simulink model "Y_Delta_Connected"  (R2018a)
settings: Solver=VariableStepAuto  StartTime=0.0  StopTime=stopTime  FixedStep=1e-8  MaxStep=1e-7  RelTol=1e-3
values from neighbouring files (symbols this model uses):
  Cp = 1/(res_w^2*Lp)    [design_code.m]
  Cs = 1/(res_w^2*Ls)    [design_code.m]
  fop = 155    [param.m]
  M = 10^6*M    [design_code.m]    (also in param.m = [p1 p1p2 p1p3 p1s1 p1s2 p1s3 ;      p1p2 p2 p2p3 p2s1 p2s2 p)
  R = [3 0 0 0 0 0 ... (first row only)    [param.m]
  R_L = Vout^2/P_o    [design_code.m]
  Vin_peak = (100)*sqrt(2)    [param.m]
libraries: powerlib x50, pePowerMeasurement x2, powerlib_meascontrol x1
settings Model: Creator=enes_  LastModifiedBy=enes_
settings SolverCC: ZeroCrossAlgorithm=Adaptive
settings DebuggingCC: MaxConsecutiveZCsMsg=none

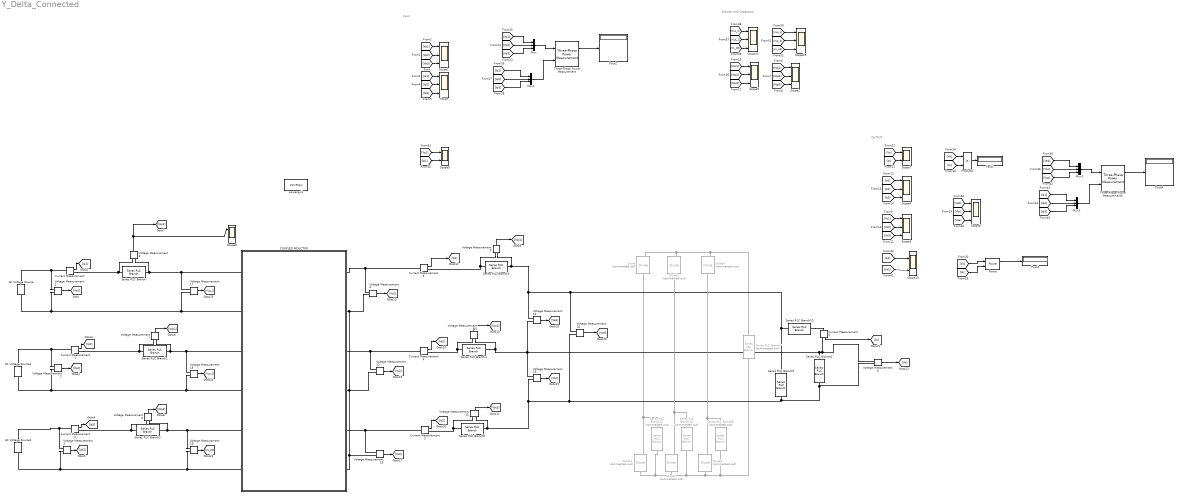
== system Y_Delta_Connected ==
  note: Inductor and Capacitors
  note: OUTPUT
  note: Input
  AC Voltage Source : powerlib/Electrical Sources/AC Voltage Source  Amplitude=Vin_peak  Phase=0  Frequency=fop*1e3  SampleTime=0  Measurements=None  BusType=swing  Pref=10e3  Qref=0  Qmin=-inf  Qmax=+inf
  AC Voltage Source1 : powerlib/Electrical Sources/AC Voltage Source  Amplitude=Vin_peak  Phase=120  Frequency=fop*1e3  SampleTime=0  Measurements=None  BusType=swing  Pref=10e3  Qref=0  Qmin=-inf  Qmax=+inf
  AC Voltage Source2 : powerlib/Electrical Sources/AC Voltage Source  Amplitude=Vin_peak  Phase=240  Frequency=fop*1e3  SampleTime=0  Measurements=None  BusType=swing  Pref=10e3  Qref=0  Qmin=-inf  Qmax=+inf
  COUPLED INDUCTOR : Subsystem
  Current Measurement{,1..6} (7 alike) : powerlib/Measurements/Current Measurement  PhasorSimulation=off  OutputType=Complex  PSBequivalent=0
  Diode{,1..5} (6 alike) : powerlib/Power Electronics/Diode  Commented=on  Ron=0.001  Lon=0  Vf=0.8  IC=0  UseSnubber=0  Rs=inf  Cs=250e-9  Measurements=on
  Mux{,1..3} (4 alike) : Mux  Inputs=3
  Pout{1..4} (4 alike) : Display
  Power : powerlib_meascontrol/Measurements/Power  Freq=fop*1e3  Vinit=[1, 0]  Iinit=[1, 0]  Ts=0
      settings: SourceProductName=Simscape Power Systems
  Product4 : Product
  Scope{,1..6,11,15} (9 alike) : Scope  NumInputPorts=3
  Scope{7..9,13} (4 alike) : Scope  NumInputPorts=2
  Series RLC Branch : powerlib/Elements/Series RLC Branch  LConnTagsString=__new0  RConnTagsString=__new0  BranchType=C  Resistance=1  Inductance=1e-3  SetiL0=off  InitialCurrent=0  Capacitance=Cp  Setx0=off  InitialVoltage=0  Measurements=None
  Series RLC Branch1 : powerlib/Elements/Series RLC Branch  LConnTagsString=__new0  RConnTagsString=__new0  BranchType=C  Resistance=1  Inductance=1e-3  SetiL0=off  InitialCurrent=0  Capacitance=Cp  Setx0=off  InitialVoltage=0  Measurements=None
  Series RLC Branch10 : powerlib/Elements/Series RLC Branch  LConnTagsString=__new0  RConnTagsString=__new0  BranchType=R  Resistance=R_L  Inductance=1e-3  SetiL0=off  InitialCurrent=0  Capacitance=9.95e-9  Setx0=off  InitialVoltage=0  Measurements=None
  Series RLC Branch15 : powerlib/Elements/Series RLC Branch  Commented=on  LConnTagsString=__new0  RConnTagsString=__new0  BranchType=R  Resistance=1e5  Inductance=1e-3  SetiL0=off  InitialCurrent=0  Capacitance=9.95e-9  Setx0=off  InitialVoltage=0  Measurements=None
  Series RLC Branch16 : powerlib/Elements/Series RLC Branch  Commented=on  LConnTagsString=__new0  RConnTagsString=__new0  BranchType=R  Resistance=1e5  Inductance=1e-3  SetiL0=off  InitialCurrent=0  Capacitance=9.95e-9  Setx0=off  InitialVoltage=0  Measurements=None
  Series RLC Branch2 : powerlib/Elements/Series RLC Branch  LConnTagsString=__new0  RConnTagsString=__new0  BranchType=C  Resistance=1  Inductance=1e-3  SetiL0=off  InitialCurrent=0  Capacitance=Cp  Setx0=off  InitialVoltage=0  Measurements=None
  Series RLC Branch3 : powerlib/Elements/Series RLC Branch  LConnTagsString=__new0  RConnTagsString=__new0  BranchType=C  Resistance=1  Inductance=1e-3  SetiL0=off  InitialCurrent=0  Capacitance=Cs  Setx0=off  InitialVoltage=0  Measurements=None
  Series RLC Branch4 : powerlib/Elements/Series RLC Branch  LConnTagsString=__new0  RConnTagsString=__new0  BranchType=C  Resistance=1  Inductance=1e-3  SetiL0=off  InitialCurrent=0  Capacitance=Cs  Setx0=off  InitialVoltage=0  Measurements=None
  Series RLC Branch5 : powerlib/Elements/Series RLC Branch  LConnTagsString=__new0  RConnTagsString=__new0  BranchType=C  Resistance=1  Inductance=1e-3  SetiL0=off  InitialCurrent=0  Capacitance=Cs  Setx0=off  InitialVoltage=0  Measurements=None
  Series RLC Branch6 : powerlib/Elements/Series RLC Branch  LConnTagsString=__new0  RConnTagsString=__new0  BranchType=R  Resistance=R_L  Inductance=1e-3  SetiL0=off  InitialCurrent=0  Capacitance=9.95e-9  Setx0=off  InitialVoltage=0  Measurements=None
  Series RLC Branch7 : powerlib/Elements/Series RLC Branch  Commented=on  LConnTagsString=__new0  RConnTagsString=__new0  BranchType=C  Resistance=30  Inductance=1e-3  SetiL0=off  InitialCurrent=0  Capacitance=1e-6  Setx0=off  InitialVoltage=0  Measurements=None
  Series RLC Branch8 : powerlib/Elements/Series RLC Branch  Commented=on  LConnTagsString=__new0  RConnTagsString=__new0  BranchType=R  Resistance=1e5  Inductance=1e-3  SetiL0=off  InitialCurrent=0  Capacitance=9.95e-9  Setx0=off  InitialVoltage=0  Measurements=None
  Series RLC Branch9 : powerlib/Elements/Series RLC Branch  LConnTagsString=__new0  RConnTagsString=__new0  BranchType=R  Resistance=R_L  Inductance=1e-3  SetiL0=off  InitialCurrent=0  Capacitance=9.95e-9  Setx0=off  InitialVoltage=0  Measurements=None
  Three-Phase Power Measurement : pePowerMeasurement/Three-Phase Power Measurement  OverrideUsingVariant=Continuous  F=fop*1e3  K=1  Seq=Negative  Ts=0
  Three-Phase Power Measurement1 : pePowerMeasurement/Three-Phase Power Measurement  OverrideUsingVariant=Continuous  F=fop*1e3  K=1  Seq=Negative  Ts=0
  Voltage Measurement{1..19} (19 alike) : powerlib/Measurements/Voltage Measurement  PhasorSimulation=off  OutputType=Complex  PSBequivalent=0
  powergui1 : powerlib/powergui  Priority=1  SimulationMode=Continuous  SampleTime=50e-6  frequency=60  Iterations=50  frequencyindice=155000  Pbase=100e6  ErrMax=1e-4  UnitsV=kV  UnitsW=MW  buscounter=0  FunctionMessages=off  echomessages=off  EnableUseOfTLC=off  CurrentSourceSwitches=off  DisableSnubberDevices=off  DisableRonSwitches=off  DisableVfSwitches=off  DisplayEquations=off  SolverType=Tustin/Backward Euler (TBE)  Interpol=off  ExternalGateDelay=off  methode=off  Ts=100  x0status=blocks  SPID=on  SwTol=0  HookPort=off  RestoreLinks=warning  ResistiveCurrentMeasurement=off  Frange=[0:2:500]  Ylog=off  Xlog=on  ShowGrid=off  save=off  variable=ZData  structure=0  ZoomFFT=off  StartTime=0.0  cycles=1  DisplayStyle=1  fundamental=60  FreqAxis=off  MaxFrequency=1000  frequencyindicesteady=1  RmsSteady=1  display=off
  wires:
  [VLp_2] -> Scope15/2
  [VL_p3] -> Scope15/3
  Voltage Measurement3/1 -> [Vp3]
  [Vsc3] -> Scope5/3
  Voltage Measurement19/1 -> [VL_p3]
  [Vsc2] -> Scope5/2
  Voltage Measurement13/1 -> [Vs3]
  [Vcp2] -> Scope2/2
  [Vcp3] -> Scope2/3
  Voltage Measurement2/1 -> [Vp2]
  [Ip2] -> Scope/2
  Voltage Measurement17/1 -> [VLp_1]
  Current Measurement2/1 -> [Ip3]
  Voltage Measurement7/1 -> [Vcp2]
  Current Measurement/1 -> [Ip1]
  [Vp1] -> Scope9/1
  [VLp_2] -> Scope11/1
  Voltage Measurement18/1 -> [VLp_2]
  Voltage Measurement11/1 -> [Vsc3]
  [Vsc1] -> Scope5/1
  [Is3] -> Scope4/3
  [VL_p3] -> Scope11/3
  Current Measurement5/1 -> [Is1]
  [Vcp1] -> Scope2/1
  [Io] -> Scope7/2
  Voltage Measurement14/1 -> [Vab]
  [Is2] -> Scope4/2
  [Vp2] -> Scope1/2
  [Vs3] -> Scope3/3
  [Vp1] -> Scope1/1
  [Vs2] -> Scope3/2
  [Vp3] -> Scope1/3
  [Vs1] -> Scope3/1
  [Ip1] -> Scope/1
  [Vo] -> Scope7/1
  Voltage Measurement9/1 -> [Vsc1]
  Current Measurement1/1 -> [Ip2]
  Voltage Measurement1/1 -> [Vp1]
  [Is1] -> Scope4/1
  [Ip3] -> Scope/3
  Voltage Measurement10/1 -> [Vsc2]
  [Ip1] -> Scope9/2
  Voltage Measurement5/1 -> [Vcp3]
  [VLp_1] -> Scope11/2
  Current Measurement4/1 -> [Is2]
  Voltage Measurement6/1 -> [Vo]
  Current Measurement3/1 -> [Is3]
  Voltage Measurement16/1 -> [Vca]
  Current Measurement6/1 -> [Io]
  Voltage Measurement12/1 -> [Vs2]
  Voltage Measurement8/1 -> Scope8/1, [Vcp1]
  Voltage Measurement4/1 -> [Vs1]
  Voltage Measurement15/1 -> [Vbc]
  [VLp_1] -> Scope15/1
  [Is1] -> Scope13/1
  [Vs1] -> Scope13/2
  [Io] -> Product4/2
  [Vo] -> Product4/1
  Product4/1 -> Pout1/1
  [Vp1] -> Mux/1
  [Vp2] -> Mux/2
  [Vp3] -> Mux/3
  [Ip2] -> Mux1/2
  [Ip1] -> Mux1/1
  [Ip3] -> Mux1/3
  Mux1/1 -> Three-Phase Power Measurement/2
  Mux/1 -> Three-Phase Power Measurement/1
  Three-Phase Power Measurement/1 -> Pout2/1
  [Vab] -> Scope6/1
  [Vca] -> Scope6/3
  [Vbc] -> Scope6/2
  [Vo] -> Power/1
  [Io] -> Power/2
  Power/1 -> Pout3/1
  [Ip1] -> Mux3/1
  [Ip3] -> Mux3/3
  [Vbc] -> Mux2/2
  [Ip2] -> Mux3/2
  [Vab] -> Mux2/1
  Mux3/1 -> Three-Phase Power Measurement1/2
  [Vca] -> Mux2/3
  Mux2/1 -> Three-Phase Power Measurement1/1
  Three-Phase Power Measurement1/1 -> Pout4/1
  connections:
  Current Measurement/LConn1 -- Voltage Measurement1/LConn1 -- AC Voltage Source/RConn1
  Diode2/RConn1 -- Series RLC Branch7/LConn1 -- Diode4/RConn1 -- Diode/RConn1
  Current Measurement4/LConn1 -- COUPLED INDUCTOR/LConn3 -- Voltage Measurement12/LConn1
  Current Measurement5/LConn1 -- Voltage Measurement4/LConn1 -- COUPLED INDUCTOR/LConn1
  Series RLC Branch/RConn1 -- Voltage Measurement8/LConn2 -- COUPLED INDUCTOR/RConn1 -- Voltage Measurement17/LConn1
  Series RLC Branch8/RConn1 -- Series RLC Branch7/RConn1 -- Series RLC Branch15/RConn1 -- Diode3/LConn1 -- Series RLC Branch16/RConn1 -- Diode1/LConn1 -- Diode5/LConn1
  Series RLC Branch4/LConn1 -- Current Measurement4/RConn1 -- Voltage Measurement10/LConn1
  Series RLC Branch1/RConn1 -- Voltage Measurement7/LConn2 -- COUPLED INDUCTOR/RConn3 -- Voltage Measurement18/LConn1
  Series RLC Branch2/LConn1 -- Current Measurement2/RConn1 -- Voltage Measurement5/LConn1
  AC Voltage Source2/RConn1 -- Current Measurement2/LConn1 -- Voltage Measurement3/LConn1
  Current Measurement1/LConn1 -- Voltage Measurement2/LConn1 -- AC Voltage Source1/RConn1
  Voltage Measurement4/LConn2 -- Voltage Measurement12/LConn2 -- COUPLED INDUCTOR/LConn4 -- Voltage Measurement13/LConn2 -- COUPLED INDUCTOR/LConn6 -- COUPLED INDUCTOR/LConn2
  Diode/LConn1 -- Series RLC Branch16/LConn1 -- Diode1/RConn1
  Series RLC Branch2/RConn1 -- COUPLED INDUCTOR/RConn5 -- Voltage Measurement19/LConn1 -- Voltage Measurement5/LConn2
  Series RLC Branch1/LConn1 -- Current Measurement1/RConn1 -- Voltage Measurement7/LConn1
  Series RLC Branch6/LConn1 -- Voltage Measurement6/LConn1 -- Current Measurement6/RConn1 -- Voltage Measurement15/LConn1 -- Voltage Measurement14/LConn2 -- Voltage Measurement10/LConn2 -- Series RLC Branch4/RConn1
  Series RLC Branch/LConn1 -- Current Measurement/RConn1 -- Voltage Measurement8/LConn1
  Series RLC Branch6/RConn1 -- Voltage Measurement16/LConn1 -- Series RLC Branch5/RConn1 -- Voltage Measurement11/LConn2 -- Voltage Measurement15/LConn2 -- Series RLC Branch9/RConn1 -- Voltage Measurement6/LConn2
  Series RLC Branch3/LConn1 -- Current Measurement5/RConn1 -- Voltage Measurement9/LConn1
  Current Measurement3/RConn1 -- Series RLC Branch5/LConn1 -- Voltage Measurement11/LConn1
  AC Voltage Source1/LConn1 -- COUPLED INDUCTOR/RConn4 -- Voltage Measurement18/LConn2 -- Voltage Measurement2/LConn2
  Voltage Measurement17/LConn2 -- COUPLED INDUCTOR/RConn2 -- AC Voltage Source/LConn1 -- Voltage Measurement1/LConn2
  Voltage Measurement19/LConn2 -- COUPLED INDUCTOR/RConn6 -- AC Voltage Source2/LConn1 -- Voltage Measurement3/LConn2
  Voltage Measurement13/LConn1 -- COUPLED INDUCTOR/LConn5 -- Current Measurement3/LConn1
  Series RLC Branch10/RConn1 -- Voltage Measurement14/LConn1 -- Voltage Measurement9/LConn2 -- Series RLC Branch3/RConn1 -- Voltage Measurement16/LConn2 -- Series RLC Branch9/LConn1
  Diode2/LConn1 -- Series RLC Branch15/LConn1 -- Diode3/RConn1
  Series RLC Branch8/LConn1 -- Diode4/LConn1 -- Diode5/RConn1
  Series RLC Branch10/LConn1 -- Current Measurement6/LConn1

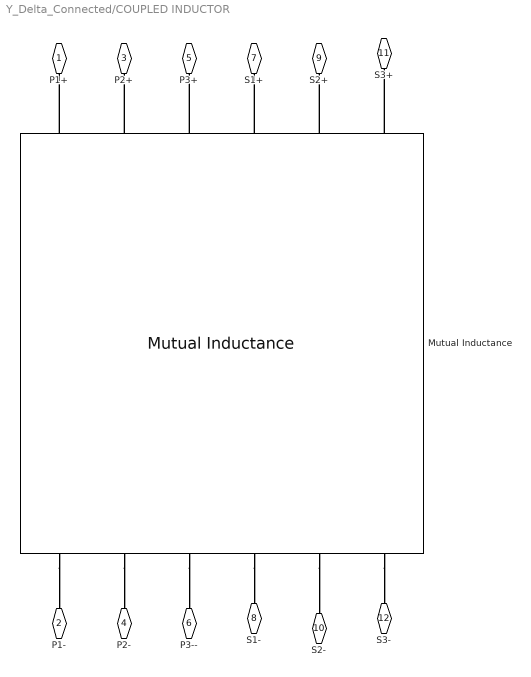
== system Y_Delta_Connected/COUPLED INDUCTOR ==
  Mutual Inductance : powerlib/Elements/Mutual Inductance  LConnTagsString=a|b|c|L4|L5|L6  RConnTagsString=A|B|C|R4|R5|R6  TypeOfMutual=Generalized mutual inductance  NumberOfWindings=6  SelfImpedance1=[1.1 1.1e-03]  SelfImpedance2=[ 1.1 1.1e-03]  ThreeWindings=on  SelfImpedance3=[ 1.1 1.1e-03]  MutualImpedance=[1.0 1.0e-03]  InductanceMatrix=M * 1e-6  ResistanceMatrix=R*0.01  Measurements=None
      settings: AttributesFormatString=\n  SourceProductName=Simscape Power Systems  SourceProductBaseCode=PS
  P1+ : PMIOPort  Side=Right
  P1- : PMIOPort  Port=2  Side=Right
  P2+ : PMIOPort  Port=3  Side=Right
  P2- : PMIOPort  Port=4  Side=Right
  P3+ : PMIOPort  Port=5  Side=Right
  P3-- : PMIOPort  Port=6  Side=Right
  S1+ : PMIOPort  Port=7  Side=Left
  S1- : PMIOPort  Port=8  Side=Left
  S2+ : PMIOPort  Port=9  Side=Left
  S2- : PMIOPort  Port=10  Side=Left
  "S3+ " : PMIOPort  Port=11  Side=Left
  "S3- " : PMIOPort  Port=12  Side=Left
  connections:
  Mutual Inductance/LConn2 -- P2-/RConn1
  Mutual Inductance/LConn5 -- S2-/RConn1
  Mutual Inductance/RConn5 -- S2+/RConn1
  Mutual Inductance/RConn4 -- S1+/RConn1
  Mutual Inductance/LConn6 -- "S3- "/RConn1
  Mutual Inductance/RConn1 -- P1+/RConn1
  Mutual Inductance/LConn1 -- P1-/RConn1
  Mutual Inductance/RConn2 -- P2+/RConn1
  Mutual Inductance/LConn4 -- S1-/RConn1
  Mutual Inductance/LConn3 -- P3--/RConn1
  Mutual Inductance/RConn3 -- P3+/RConn1
  Mutual Inductance/RConn6 -- "S3+ "/RConn1
